simulink model "GolfSwing"  (R2024b)
settings: Solver=VariableStepAuto  StartTime=0.0  StopTime=StopTime  MaxStep=0.001  RelTol=1e-3
PreLoadFcn:
  | cd(matlabdrive);
  | cd '2DModel';
PostLoadFcn:
  | %run SCRIPT_mdlWksGenerate.m;
  | mdlWks=get_param('GolfSwing','ModelWorkspace');
  | mdlWks.DataSource = 'MAT-File';
  | mdlWks.FileName = 'ModelInputs.mat';
  | mdlWks.reload;
model workspace: external: MAT-File ModelInputs.mat (data not in the file)
undefined symbols (not defined in the file or in its folder): GlobalGain, HipConstant, HipDampening, HipTimeGain, KillDampFinalValue, KillDampInitialValue, KillswitchFinalValue, KillswitchInitialValue, KillswitchStepTime, LElbowConstant, LElbowDampening, LElbowTimeGain, LScapConstant, LScapDampening, LScapPositionGain, LScapTimeGain, LShoulderConstant, LShoulderDampening, LShoulderTimeGain, LWristConstant, LWristDampening, LWristTimeGain, RElbowConstant, RElbowDampening, RElbowTimeGain, RScapConstant, RScapDampening, RScapPositionGain, RScapTimeGain, RShoulderConstant, RShoulderDampening, RShoulderTimeGain, RWristConstant, RWristDampening, RWristTimeGain, TorsoConstant, TorsoDampening, TorsoPositionGain, TorsoTimeGain, WristGain, X, Y, Z
libraries: nesl_utility x207, sm_lib x106, matrix_library x11, simulink_extras x2, simulink x1
(part 5 of 6)

== system GolfSwing/Right Upper Arm MOF ==
  RS Global Position : Inport
  RE Global Position : Inport  Port=2
  RSonRArmFGlobalIn : Inport  Port=3
  RSonRArmTGlobalIn : Inport  Port=4
  RForearmonRArmFGlobalIn : Inport  Port=5
  RForearmonRArmTGlobalIn : Inport  Port=6
  R Vector Elbow Force on Right Arm : Sum  Inputs=-+
  R Vector Shoulder Force on Right Arm : Sum  Inputs=-+
  RElbowonRArmMOFGlobal : matrix_library/Cross Product
  RElbowonRArmMOFLocal : Product  Multiplication=Matrix(*)
  RSAngularImpulseonArm : Integrator
  RShoulderonRArmMOFGlobal : matrix_library/Cross Product
  RShoulderonRArmMOFLocal : Product  Multiplication=Matrix(*)
  RUACOM : sm_lib/Body Elements/Inertia Sensor  SensorExtent=BodyGroup  SpanWeldJoints=off  ExcludeGroundedBodies=off  MeasurementFrame=World  SenseMass=off  SenseCenterOfMass=on  SenseInertiaMatrix=off  SenseCenteredInertiaMatrix=off  SensePrincipalInertiaMatrix=off  SenseRotationMatrix=off  GraphicType=None  PrincipalInertiaFrameSize=20  GraphicVisPropType=SimpleVisualProperties  GraphicDiffuseColor=[0.5 0.5 0.5]  GraphicOpacity=1  GraphicSpecularColor=[0.5 0.5 0.5 1.0]  GraphicAmbientColor=[0.15 0.15 0.15 1.0]  GraphicEmissiveColor=[0.0 0.0 0.0 1.0]  GraphicShininess=75
  Right Upper Arm COM : nesl_utility/PS-Simulink Converter  PhysicalDomain=network_engine_domain  SubClassName=ps_output  LeftPortType=input  RightPortType=output  PseudoPeriodic=off  Frequencies=[]  VectorFormat=1-D array  Unit=inherit  AffineConversion=off
  Rotation Transform Right Arm : nesl_utility/PS-Simulink Converter  PhysicalDomain=network_engine_domain  SubClassName=ps_output  LeftPortType=input  RightPortType=output  PseudoPeriodic=off  Frequencies=[]  VectorFormat=1-D array  Unit=inherit  AffineConversion=off
  SumofMomentsRArmLocal : Product  Multiplication=Matrix(*)
  SumofMomentsRSonRArm : Sum
  SumofMomentsRightArmGlobal : Sum  Inputs=++++
  Transform Sensor : sm_lib/Frames and Transforms/Transform Sensor  MeasurementFrame=World  RotationSequence=XYX  SenseAngle=off  SenseAxis=off  SenseQ=off  SenseR=on  SenseRotationSequence=off  SenseOmegaX=off  SenseOmegaY=off  SenseOmegaZ=off  SenseOmega=off  SenseQDot=off  SenseRDot=off  SenseRotationSequenceDot=off  SenseAlphaX=off  SenseAlphaY=off  SenseAlphaZ=off  SenseAlpha=off  SenseQDDot=off  SenseRDDot=off  SenseX=off  SenseY=off  SenseZ=off  SenseXYZ=off  SenseRad=off  SenseAzim=off  SenseDist=off  SenseInc=off  SenseXDot=off  SenseYDot=off  SenseZDot=off  SenseXYZDot=off  SenseRadDot=off  SenseAzimDot=off  SenseDistDot=off  SenseIncDot=off  SenseXDDot=off  SenseYDDot=off  SenseZDDot=off  SenseXYZDDot=off  SenseRadDDot=off  SenseAzimDDot=off  SenseDistDDot=off  SenseIncDDot=off
  World Frame : sm_lib/Frames and Transforms/World Frame
  RightUpper  Arm : PMIOPort  Side=Left
  wires:
  Right Upper Arm COM/1 -> R Vector Elbow Force on Right Arm/1, R Vector Shoulder Force on Right Arm/1  "RUpperArmCOM"
  RS Global Position/1 -> R Vector Shoulder Force on Right Arm/2
  RE Global Position/1 -> R Vector Elbow Force on Right Arm/2
  RSonRArmFGlobalIn/1 -> RShoulderonRArmMOFGlobal/2
  R Vector Elbow Force on Right Arm/1 -> RElbowonRArmMOFGlobal/1
  RForearmonRArmTGlobalIn/1 -> SumofMomentsRightArmGlobal/4
  RForearmonRArmFGlobalIn/1 -> RElbowonRArmMOFGlobal/2
  R Vector Shoulder Force on Right Arm/1 -> RShoulderonRArmMOFGlobal/1
  SumofMomentsRightArmGlobal/1 -> SumofMomentsRArmLocal/2  "SumofMomentsRightArmGlobal"
  RElbowonRArmMOFGlobal/1 -> RElbowonRArmMOFLocal/2, SumofMomentsRightArmGlobal/2  "RElbowonRArmMOFGlobal"
  Rotation Transform Right Arm/1 -> SumofMomentsRArmLocal/1, RElbowonRArmMOFLocal/1, RShoulderonRArmMOFLocal/1
  RShoulderonRArmMOFGlobal/1 -> SumofMomentsRightArmGlobal/1, SumofMomentsRSonRArm/2, RShoulderonRArmMOFLocal/2  "RShoulderonRArmMOFGlobal"
  SumofMomentsRSonRArm/1 -> RSAngularImpulseonArm/1  "SumofMomentsRSonRArm"
  RSonRArmTGlobalIn/1 -> SumofMomentsRSonRArm/1, SumofMomentsRightArmGlobal/3
  connections:
  RUACOM/LConn1 -- Transform Sensor/LConn1 -- RightUpper  Arm/RConn1
  Right Upper Arm COM/LConn1 -- RUACOM/RConn1
  Transform Sensor/RConn1 -- World Frame/RConn1
  Rotation Transform Right Arm/LConn1 -- Transform Sensor/RConn2

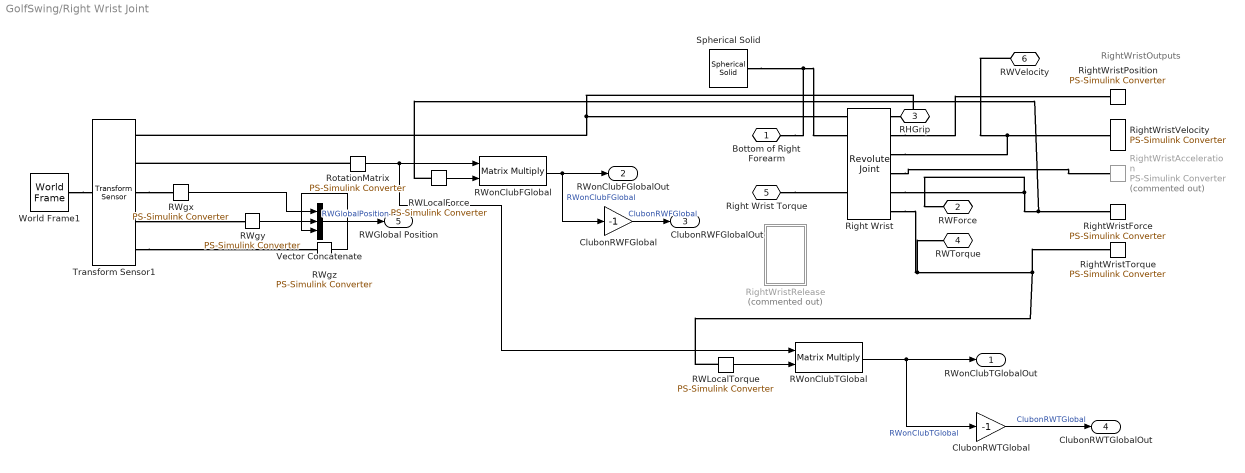
== system GolfSwing/Right Wrist Joint ==
  note: RightWristOutputs
  ClubonRWFGlobal : Gain  Gain=-1
  ClubonRWTGlobal : Gain  Gain=-1
  RWLocalForce : nesl_utility/PS-Simulink Converter  PhysicalDomain=network_engine_domain  SubClassName=ps_output  LeftPortType=input  RightPortType=output  PseudoPeriodic=off  Frequencies=[]  VectorFormat=1-D array  Unit=inherit  AffineConversion=off
  RWLocalTorque : nesl_utility/PS-Simulink Converter  PhysicalDomain=network_engine_domain  SubClassName=ps_output  LeftPortType=input  RightPortType=output  PseudoPeriodic=off  Frequencies=[]  VectorFormat=1-D array  Unit=inherit  AffineConversion=off
  RWgx : nesl_utility/PS-Simulink Converter  PhysicalDomain=network_engine_domain  SubClassName=ps_output  LeftPortType=input  RightPortType=output  PseudoPeriodic=off  Frequencies=[]  VectorFormat=1-D array  Unit=inherit  AffineConversion=off
  RWgy : nesl_utility/PS-Simulink Converter  PhysicalDomain=network_engine_domain  SubClassName=ps_output  LeftPortType=input  RightPortType=output  PseudoPeriodic=off  Frequencies=[]  VectorFormat=1-D array  Unit=inherit  AffineConversion=off
  RWgz : nesl_utility/PS-Simulink Converter  PhysicalDomain=network_engine_domain  SubClassName=ps_output  LeftPortType=input  RightPortType=output  PseudoPeriodic=off  Frequencies=[]  VectorFormat=1-D array  Unit=inherit  AffineConversion=off
  RWonClubFGlobal : Product  Multiplication=Matrix(*)
  RWonClubTGlobal : Product  Multiplication=Matrix(*)
  Right Wrist : sm_lib/Joints/Revolute Joint  JointMode=Normal  CompositeWrenchDir=BaseOnFollower  CompositeWrenchFrame=FollowerFrame  SenseConstraintForce=off  SenseConstraintTorque=off  SenseTotalForce=on  SenseTotalTorque=on  PositionTargetSpecify=off  PositionTargetPriority=Low  PositionTargetValue=70  PositionTargetValueUnits=deg  VelocityTargetSpecify=off  VelocityTargetPriority=Low  VelocityTargetValue=0  VelocityTargetValueUnits=deg/s  EquilibriumPosition=0  EquilibriumPositionUnits=deg  SpringStiffness=0  SpringStiffnessUnits=N*m/deg  DampingCoefficient=0  DampingCoefficientUnits=N*m/(deg/s)  LowerLimitSpecify=off  LowerLimitBound=-90  LowerLimitBoundUnits=deg  LowerLimitStiffness=1e4  LowerLimitStiffnessUnits=N*m/deg  LowerLimitDamping=10  LowerLimitDampingUnits=N*m/(deg/s)  LowerLimitTransitionRegionWidth=0.1  LowerLimitTransitionRegionWidthUnits=deg  UpperLimitSpecify=off  UpperLimitBound=90  UpperLimitBoundUnits=deg  UpperLimitStiffness=1e4  UpperLimitStiffnessUnits=N*m/deg  UpperLimitDamping=10  UpperLimitDampingUnits=N*m/(deg/s)  UpperLimitTransitionRegionWidth=0.1  UpperLimitTransitionRegionWidthUnits=deg  TorqueActuationMode=InputTorque  MotionActuationMode=ComputedMotion  SensePosition=on  SenseVelocity=on  SenseAcceleration=on  SenseTorqueForce=off  SenseLowerLimitTorqueForce=off  SenseUpperLimitTorqueForce=off
      settings: LogSimulationData=on
  RightWristAcceleration : nesl_utility/PS-Simulink Converter  Commented=on  PhysicalDomain=network_engine_domain  SubClassName=ps_output  LeftPortType=input  RightPortType=output  PseudoPeriodic=off  Frequencies=[]  VectorFormat=1-D array  Unit=inherit  AffineConversion=off
  RightWristForce : nesl_utility/PS-Simulink Converter  PhysicalDomain=network_engine_domain  SubClassName=ps_output  LeftPortType=input  RightPortType=output  PseudoPeriodic=off  Frequencies=[]  VectorFormat=1-D array  Unit=inherit  AffineConversion=off
  RightWristPosition : nesl_utility/PS-Simulink Converter  PhysicalDomain=network_engine_domain  SubClassName=ps_output  LeftPortType=input  RightPortType=output  PseudoPeriodic=off  Frequencies=[]  VectorFormat=1-D array  Unit=inherit  AffineConversion=off
  RightWristRelease : Subsystem  Commented=on
  RightWristTorque : nesl_utility/PS-Simulink Converter  PhysicalDomain=network_engine_domain  SubClassName=ps_output  LeftPortType=input  RightPortType=output  PseudoPeriodic=off  Frequencies=[]  VectorFormat=1-D array  Unit=inherit  AffineConversion=off
  RightWristVelocity : nesl_utility/PS-Simulink Converter  PhysicalDomain=network_engine_domain  SubClassName=ps_output  LeftPortType=input  RightPortType=output  PseudoPeriodic=off  Frequencies=[]  VectorFormat=1-D array  Unit=inherit  AffineConversion=off
  RotationMatrix : nesl_utility/PS-Simulink Converter  PhysicalDomain=network_engine_domain  SubClassName=ps_output  LeftPortType=input  RightPortType=output  PseudoPeriodic=off  Frequencies=[]  VectorFormat=1-D array  Unit=inherit  AffineConversion=off
  Spherical Solid : sm_lib/Body Elements/Spherical Solid  SphereRadius=2  SphereRadiusUnits=in  ExportEntireGeometry=off  InertiaType=CalculateFromGeometry  BasedOnType=Density  Density=0  DensityUnits=kg/m^3  Mass=1  MassUnits=kg  CenterOfMass=[0 0 0]  CenterOfMassUnits=m  MomentsOfInertia=[1 1 1]  MomentsOfInertiaUnits=kg*m^2  ProductsOfInertia=[0 0 0]  ProductsOfInertiaUnits=kg*m^2  GraphicType=FromGeometry  MarkerShape=Sphere  MarkerSize=10  GraphicVisPropType=SimpleVisualProperties  GraphicDiffuseColor=[1.0 0.8 0.4]  GraphicOpacity=1  GraphicSpecularColor=[0.5 0.5 0.5 1.0]  GraphicAmbientColor=[0.15 0.15 0.15 1.0]  GraphicEmissiveColor=[0.0 0.0 0.0 1.0]  GraphicShininess=75  DoExposeReferenceFrame=on  SerializedFrames=<Frames/>
  Transform Sensor1 : sm_lib/Frames and Transforms/Transform Sensor  MeasurementFrame=World  RotationSequence=XYX  SenseAngle=off  SenseAxis=off  SenseQ=off  SenseR=on  SenseRotationSequence=off  SenseOmegaX=off  SenseOmegaY=off  SenseOmegaZ=off  SenseOmega=off  SenseQDot=off  SenseRDot=off  SenseRotationSequenceDot=off  SenseAlphaX=off  SenseAlphaY=off  SenseAlphaZ=off  SenseAlpha=off  SenseQDDot=off  SenseRDDot=off  SenseX=on  SenseY=on  SenseZ=on  SenseXYZ=off  SenseRad=off  SenseAzim=off  SenseDist=off  SenseInc=off  SenseXDot=off  SenseYDot=off  SenseZDot=off  SenseXYZDot=off  SenseRadDot=off  SenseAzimDot=off  SenseDistDot=off  SenseIncDot=off  SenseXDDot=off  SenseYDDot=off  SenseZDDot=off  SenseXYZDDot=off  SenseRadDDot=off  SenseAzimDDot=off  SenseDistDDot=off  SenseIncDDot=off
  Vector Concatenate : Concatenate  NumInputs=3
  World Frame1 : sm_lib/Frames and Transforms/World Frame
  Bottom of Right Forearm : PMIOPort  Side=Left
  RWForce : PMIOPort  Port=2  Side=Right
  RHGrip : PMIOPort  Port=3  Side=Right
  RWTorque : PMIOPort  Port=4  Side=Right
  Right Wrist Torque : PMIOPort  Port=5  Side=Right
  RWVelocity : PMIOPort  Port=6  Side=Right
  RWonClubTGlobalOut : Outport
  RWonClubFGlobalOut : Outport  Port=2
  ClubonRWFGlobalOut : Outport  Port=3
  ClubonRWTGlobalOut : Outport  Port=4
  RWGlobal Position : Outport  Port=5
  wires:
  RWLocalForce/1 -> RWonClubFGlobal/2
  RotationMatrix/1 -> RWonClubTGlobal/1, RWonClubFGlobal/1
  RWLocalTorque/1 -> RWonClubTGlobal/2
  ClubonRWFGlobal/1 -> ClubonRWFGlobalOut/1  "ClubonRWFGlobal"
  RWonClubFGlobal/1 -> ClubonRWFGlobal/1, RWonClubFGlobalOut/1  "RWonClubFGlobal"
  RWonClubTGlobal/1 -> ClubonRWTGlobal/1, RWonClubTGlobalOut/1  "RWonClubTGlobal"
  ClubonRWTGlobal/1 -> ClubonRWTGlobalOut/1  "ClubonRWTGlobal"
  RWgx/1 -> Vector Concatenate/1
  RWgz/1 -> Vector Concatenate/3
  Vector Concatenate/1 -> RWGlobal Position/1  "RWGlobalPosition"
  RWgy/1 -> Vector Concatenate/2
  connections:
  Bottom of Right Forearm/RConn1 -- Spherical Solid/RConn1 -- Right Wrist/LConn1
  Right Wrist/RConn1 -- Transform Sensor1/RConn1 -- RHGrip/RConn1
  Right Wrist Torque/RConn1 -- Right Wrist/LConn2
  RotationMatrix/LConn1 -- Transform Sensor1/RConn2
  World Frame1/RConn1 -- Transform Sensor1/LConn1
  Transform Sensor1/RConn4 -- RWgy/LConn1
  Transform Sensor1/RConn5 -- RWgz/LConn1
  Transform Sensor1/RConn3 -- RWgx/LConn1
  Right Wrist/RConn3 -- RightWristVelocity/LConn1 -- RWVelocity/RConn1
  Right Wrist/RConn2 -- RightWristPosition/LConn1
  Right Wrist/RConn5 -- RightWristForce/LConn1 -- RWLocalForce/LConn1 -- RWForce/RConn1
  Right Wrist/RConn6 -- RightWristTorque/LConn1 -- RWLocalTorque/LConn1 -- RWTorque/RConn1
  Right Wrist/RConn4 -- RightWristAcceleration/LConn1

== system GolfSwing/TorsoOutputs ==
  TorsoAcceleration : nesl_utility/PS-Simulink Converter  Commented=on  PhysicalDomain=network_engine_domain  SubClassName=ps_output  LeftPortType=input  RightPortType=output  PseudoPeriodic=off  Frequencies=[]  VectorFormat=1-D array  Unit=inherit  AffineConversion=off
  TorsoForce : nesl_utility/PS-Simulink Converter  PhysicalDomain=network_engine_domain  SubClassName=ps_output  LeftPortType=input  RightPortType=output  PseudoPeriodic=off  Frequencies=[]  VectorFormat=1-D array  Unit=inherit  AffineConversion=off
  TorsoPosition : nesl_utility/PS-Simulink Converter  PhysicalDomain=network_engine_domain  SubClassName=ps_output  LeftPortType=input  RightPortType=output  PseudoPeriodic=off  Frequencies=[]  VectorFormat=1-D array  Unit=inherit  AffineConversion=off
  TorsoTorque : nesl_utility/PS-Simulink Converter  PhysicalDomain=network_engine_domain  SubClassName=ps_output  LeftPortType=input  RightPortType=output  PseudoPeriodic=off  Frequencies=[]  VectorFormat=1-D array  Unit=inherit  AffineConversion=off
  TorsoVelocity : nesl_utility/PS-Simulink Converter  PhysicalDomain=network_engine_domain  SubClassName=ps_output  LeftPortType=input  RightPortType=output  PseudoPeriodic=off  Frequencies=[]  VectorFormat=1-D array  Unit=inherit  AffineConversion=off
  TorsPosition : PMIOPort  Side=Left
  TorsVel : PMIOPort  Port=2  Side=Left
  TorsAccel : PMIOPort  Port=3  Side=Left
  TorsForce : PMIOPort  Port=4  Side=Left
  TorsTorque : PMIOPort  Port=5  Side=Left
  connections:
  TorsForce/RConn1 -- TorsoForce/LConn1
  TorsVel/RConn1 -- TorsoVelocity/LConn1
  TorsTorque/RConn1 -- TorsoTorque/LConn1
  TorsAccel/RConn1 -- TorsoAcceleration/LConn1
  TorsPosition/RConn1 -- TorsoPosition/LConn1

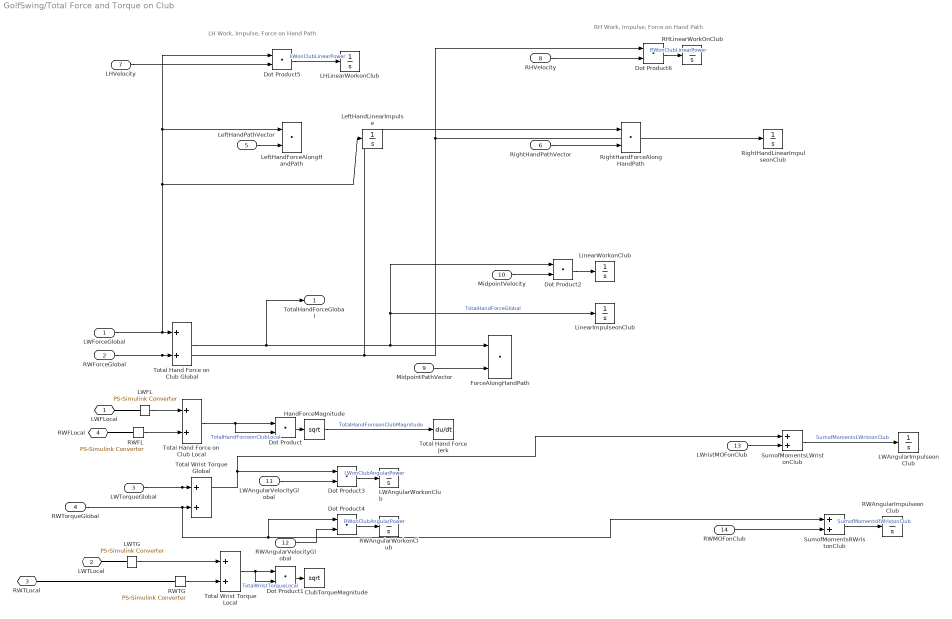
== system GolfSwing/Total Force and Torque on Club ==
  note: RH Work, Impulse, Force on Hand Path
  note: LH Work, Impulse, Force on Hand Path
  LWForceGlobal : Inport
  RWForceGlobal : Inport  Port=2
  LWTorqueGlobal : Inport  Port=3
  RWTorqueGlobal : Inport  Port=4
  LeftHandPathVector : Inport  Port=5
  RightHandPathVector : Inport  Port=6
  LHVelocity : Inport  Port=7
  RHVelocity : Inport  Port=8
  MidpointPathVector : Inport  Port=9
  MidpointVelocity : Inport  Port=10
  LWAngularVelocityGlobal : Inport  Port=11
  RWAngularVelocityGlobal : Inport  Port=12
  LWristMOFonClub : Inport  Port=13
  RWMOFonClub : Inport  Port=14
  ClubTorqueMagnitude : Sqrt
  Dot Product{,1..6} (7 alike) : DotProduct  OutDataTypeStr=Inherit: Inherit via internal rule
  ForceAlongHandPath : DotProduct  OutDataTypeStr=Inherit: Inherit via internal rule
  HandForceMagnitude : Sqrt
  LHLinearWorkonClub : Integrator
  LWAngularImpulseonClub : Integrator
  LWAngularWorkonClub : Integrator
  LWFL : nesl_utility/PS-Simulink Converter  PhysicalDomain=network_engine_domain  SubClassName=ps_output  LeftPortType=input  RightPortType=output  PseudoPeriodic=off  Frequencies=[]  VectorFormat=1-D array  Unit=inherit  AffineConversion=off
  LWTG : nesl_utility/PS-Simulink Converter  PhysicalDomain=network_engine_domain  SubClassName=ps_output  LeftPortType=input  RightPortType=output  PseudoPeriodic=off  Frequencies=[]  VectorFormat=1-D array  Unit=inherit  AffineConversion=off
  LeftHandForceAlongHandPath : DotProduct  OutDataTypeStr=Inherit: Inherit via internal rule
  LeftHandLinearImpulse : Integrator
  LinearImpulseonClub : Integrator
  LinearWorkonClub : Integrator
  RHLinearWorkOnClub : Integrator
  RWAngularImpulseonClub : Integrator
  RWAngularWorkonClub : Integrator
  RWFL : nesl_utility/PS-Simulink Converter  PhysicalDomain=network_engine_domain  SubClassName=ps_output  LeftPortType=input  RightPortType=output  PseudoPeriodic=off  Frequencies=[]  VectorFormat=1-D array  Unit=inherit  AffineConversion=off
  RWTG : nesl_utility/PS-Simulink Converter  PhysicalDomain=network_engine_domain  SubClassName=ps_output  LeftPortType=input  RightPortType=output  PseudoPeriodic=off  Frequencies=[]  VectorFormat=1-D array  Unit=inherit  AffineConversion=off
  RightHandForceAlongHandPath : DotProduct  OutDataTypeStr=Inherit: Inherit via internal rule
  RightHandLinearImpulseonClub : Integrator
  SumofMomentsLWristonClub : Sum
  SumofMomentsRWristonClub : Sum
  Total Hand Force Jerk : Derivative
  Total Hand Force on Club Global : Sum
  Total Hand Force on Club Local : Sum
  Total Wrist Torque Global : Sum
  Total Wrist Torque Local : Sum
  LWFLocal : PMIOPort  Side=Left
  LWTLocal : PMIOPort  Port=2  Side=Left
  RWTLocal : PMIOPort  Port=3  Side=Left
  RWFLocal : PMIOPort  Port=4  Side=Left
  TotalHandForceGlobal : Outport
  wires:
  RWFL/1 -> Total Hand Force on Club Local/2
  Total Wrist Torque Local/1 -> Dot Product1/1, Dot Product1/2  "TotalWristTorqueLocal"
  LWFL/1 -> Total Hand Force on Club Local/1
  Dot Product/1 -> HandForceMagnitude/1
  Dot Product1/1 -> ClubTorqueMagnitude/1
  Total Hand Force on Club Local/1 -> Dot Product/2, Dot Product/1  "TotalHandForceonClubLocal"
  Total Hand Force on Club Global/1 -> Dot Product2/1, LinearImpulseonClub/1, ForceAlongHandPath/1, TotalHandForceGlobal/1  "TotalHandForceGlobal"
  LWTG/1 -> Total Wrist Torque Local/1
  RWTG/1 -> Total Wrist Torque Local/2
  LWTorqueGlobal/1 -> Dot Product3/1, SumofMomentsLWristonClub/1, Total Wrist Torque Global/1
  MidpointPathVector/1 -> ForceAlongHandPath/2
  Dot Product2/1 -> LinearWorkonClub/1
  MidpointVelocity/1 -> Dot Product2/2
  Dot Product3/1 -> LWAngularWorkonClub/1  "LWonClubAngularPower"
  LWAngularVelocityGlobal/1 -> Dot Product3/2
  Dot Product4/1 -> RWAngularWorkonClub/1  "RWonClubAngularPower"
  RWAngularVelocityGlobal/1 -> Dot Product4/2
  RWTorqueGlobal/1 -> Dot Product4/1, SumofMomentsRWristonClub/1, Total Wrist Torque Global/2
  SumofMomentsLWristonClub/1 -> LWAngularImpulseonClub/1  "SumofMomentsLWristonClub"
  SumofMomentsRWristonClub/1 -> RWAngularImpulseonClub/1  "SumofMomentsRWristonClub"
  LWristMOFonClub/1 -> SumofMomentsLWristonClub/2
  RWMOFonClub/1 -> SumofMomentsRWristonClub/2
  LHVelocity/1 -> Dot Product5/2
  LWForceGlobal/1 -> Dot Product5/1, LeftHandForceAlongHandPath/1, LeftHandLinearImpulse/1, Total Hand Force on Club Global/1
  Dot Product5/1 -> LHLinearWorkonClub/1  "LWonClubLinearPower"
  LeftHandPathVector/1 -> LeftHandForceAlongHandPath/2
  RHVelocity/1 -> Dot Product6/2
  RWForceGlobal/1 -> RightHandLinearImpulseonClub/1, Dot Product6/1, RightHandForceAlongHandPath/1, Total Hand Force on Club Global/2
  Dot Product6/1 -> RHLinearWorkOnClub/1  "RWonClubLinearPower"
  RightHandPathVector/1 -> RightHandForceAlongHandPath/2
  HandForceMagnitude/1 -> Total Hand Force Jerk/1  "TotalHandForceonClubMagnitude"
  connections:
  LWFLocal/RConn1 -- LWFL/LConn1
  RWFLocal/RConn1 -- RWFL/LConn1
  LWTG/LConn1 -- LWTLocal/RConn1
  RWTLocal/RConn1 -- RWTG/LConn1

== system GolfSwing/Club/ButtGlobal ==
  Buttx : nesl_utility/PS-Simulink Converter  PhysicalDomain=network_engine_domain  SubClassName=ps_output  LeftPortType=input  RightPortType=output  PseudoPeriodic=off  Frequencies=[]  VectorFormat=1-D array  Unit=inherit  AffineConversion=off
  Butty : nesl_utility/PS-Simulink Converter  PhysicalDomain=network_engine_domain  SubClassName=ps_output  LeftPortType=input  RightPortType=output  PseudoPeriodic=off  Frequencies=[]  VectorFormat=1-D array  Unit=inherit  AffineConversion=off
  Buttz : nesl_utility/PS-Simulink Converter  PhysicalDomain=network_engine_domain  SubClassName=ps_output  LeftPortType=input  RightPortType=output  PseudoPeriodic=off  Frequencies=[]  VectorFormat=1-D array  Unit=inherit  AffineConversion=off
  Transform Sensor : sm_lib/Frames and Transforms/Transform Sensor  MeasurementFrame=World  RotationSequence=XYX  SenseAngle=off  SenseAxis=off  SenseQ=off  SenseR=off  SenseRotationSequence=off  SenseOmegaX=off  SenseOmegaY=off  SenseOmegaZ=off  SenseOmega=off  SenseQDot=off  SenseRDot=off  SenseRotationSequenceDot=off  SenseAlphaX=off  SenseAlphaY=off  SenseAlphaZ=off  SenseAlpha=off  SenseQDDot=off  SenseRDDot=off  SenseX=on  SenseY=on  SenseZ=on  SenseXYZ=off  SenseRad=off  SenseAzim=off  SenseDist=off  SenseInc=off  SenseXDot=off  SenseYDot=off  SenseZDot=off  SenseXYZDot=off  SenseRadDot=off  SenseAzimDot=off  SenseDistDot=off  SenseIncDot=off  SenseXDDot=off  SenseYDDot=off  SenseZDDot=off  SenseXYZDDot=off  SenseRadDDot=off  SenseAzimDDot=off  SenseDistDDot=off  SenseIncDDot=off
  Conn1 : PMIOPort  Side=Right
  Conn2 : PMIOPort  Port=2  Side=Left
  connections:
  Buttx/LConn1 -- Transform Sensor/RConn2
  Buttz/LConn1 -- Transform Sensor/RConn4
  Butty/LConn1 -- Transform Sensor/RConn3
  Transform Sensor/LConn1 -- Conn2/RConn1
  Transform Sensor/RConn1 -- Conn1/RConn1

== system GolfSwing/Club/CHGlobal ==
  AoA Calculation : Subsystem
  CHS (m/s) : Subsystem
  CHSmph : Gain  Gain=2.23694
  CHvx : nesl_utility/PS-Simulink Converter  PhysicalDomain=network_engine_domain  SubClassName=ps_output  LeftPortType=input  RightPortType=output  PseudoPeriodic=off  Frequencies=[]  VectorFormat=1-D array  Unit=inherit  AffineConversion=off
  CHvy : nesl_utility/PS-Simulink Converter  PhysicalDomain=network_engine_domain  SubClassName=ps_output  LeftPortType=input  RightPortType=output  PseudoPeriodic=off  Frequencies=[]  VectorFormat=1-D array  Unit=inherit  AffineConversion=off
  CHvz : nesl_utility/PS-Simulink Converter  PhysicalDomain=network_engine_domain  SubClassName=ps_output  LeftPortType=input  RightPortType=output  PseudoPeriodic=off  Frequencies=[]  VectorFormat=1-D array  Unit=inherit  AffineConversion=off
  CHx : nesl_utility/PS-Simulink Converter  PhysicalDomain=network_engine_domain  SubClassName=ps_output  LeftPortType=input  RightPortType=output  PseudoPeriodic=off  Frequencies=[]  VectorFormat=1-D array  Unit=inherit  AffineConversion=off
  CHy : nesl_utility/PS-Simulink Converter  PhysicalDomain=network_engine_domain  SubClassName=ps_output  LeftPortType=input  RightPortType=output  PseudoPeriodic=off  Frequencies=[]  VectorFormat=1-D array  Unit=inherit  AffineConversion=off
  CHz : nesl_utility/PS-Simulink Converter  PhysicalDomain=network_engine_domain  SubClassName=ps_output  LeftPortType=input  RightPortType=output  PseudoPeriodic=off  Frequencies=[]  VectorFormat=1-D array  Unit=inherit  AffineConversion=off
  ClubheadPathUnitVector : Mux  Inputs=3
  Constant : Constant  Value=0
  Filtering Block : Subsystem  Commented=on
  MinMax Running Resettable : simulink/Math Operations/MinMax Running Resettable  Function=max  vinit=0.0
  Path Calculation : Subsystem
  Transform Sensor : sm_lib/Frames and Transforms/Transform Sensor  MeasurementFrame=World  RotationSequence=XYX  SenseAngle=off  SenseAxis=off  SenseQ=off  SenseR=off  SenseRotationSequence=off  SenseOmegaX=off  SenseOmegaY=off  SenseOmegaZ=off  SenseOmega=off  SenseQDot=off  SenseRDot=off  SenseRotationSequenceDot=off  SenseAlphaX=off  SenseAlphaY=off  SenseAlphaZ=off  SenseAlpha=off  SenseQDDot=off  SenseRDDot=off  SenseX=on  SenseY=on  SenseZ=on  SenseXYZ=off  SenseRad=off  SenseAzim=off  SenseDist=off  SenseInc=off  SenseXDot=on  SenseYDot=on  SenseZDot=on  SenseXYZDot=off  SenseRadDot=off  SenseAzimDot=off  SenseDistDot=off  SenseIncDot=off  SenseXDDot=off  SenseYDDot=off  SenseZDDot=off  SenseXYZDDot=off  SenseRadDDot=off  SenseAzimDDot=off  SenseDistDDot=off  SenseIncDDot=off
  UnitVectorX : Product  Inputs=*/
  UnitVectorY : Product  Inputs=*/
  UnitVectorZ : Product  Inputs=*/
  Clubhead : PMIOPort  Side=Right
  Global : PMIOPort  Port=2  Side=Left
  ClubPathUV : Outport
  CHSMPS : Outport  Port=2
  wires:
  CHvy/1 -> Path Calculation/1(Vy), AoA Calculation/2(Vy), UnitVectorY/1, CHS (m/s)/2(In2)  "CHvy"
  CHvx/1 -> AoA Calculation/1(Vx), Path Calculation/2(Vx), UnitVectorX/1, CHS (m/s)/1(In1)  "CHvx"
  CHvz/1 -> CHS (m/s)/3(In3), AoA Calculation/3(Vz), UnitVectorZ/1  "CHvz"
  UnitVectorZ/1 -> ClubheadPathUnitVector/3
  UnitVectorY/1 -> ClubheadPathUnitVector/2
  CHS (m/s)/1(ClubPathUV1) -> CHSMPS/1, CHSmph/1, UnitVectorZ/2, UnitVectorY/2, UnitVectorX/2  "CHSmpersec"
  UnitVectorX/1 -> ClubheadPathUnitVector/1
  ClubheadPathUnitVector/1 -> ClubPathUV/1  "ClubPathUV"
  CHSmph/1 -> MinMax Running Resettable/1, Filtering Block/1(CHS (mph))  "CHS (mph)"
  Constant/1 -> MinMax Running Resettable/2
  connections:
  CHx/LConn1 -- Transform Sensor/RConn2
  CHz/LConn1 -- Transform Sensor/RConn4
  CHvz/LConn1 -- Transform Sensor/RConn7
  CHy/LConn1 -- Transform Sensor/RConn3
  Transform Sensor/RConn5 -- CHvx/LConn1
  CHvy/LConn1 -- Transform Sensor/RConn6
  Transform Sensor/LConn1 -- Global/RConn1
  Transform Sensor/RConn1 -- Clubhead/RConn1

== system GolfSwing/Club/Clubhead Air Resistance Calculator ==
  CHSmps : Inport
  ClubPathUV : Inport  Port=2
  Add : Sum  Inputs=+++
  Air Resistance : sm_lib/Forces and Torques/External Force and Torque  EnableForceX=off  EnableForceY=off  EnableForceZ=off  EnableForce=on  ForceResolutionFrame=World  EnableTorqueX=off  EnableTorqueY=off  EnableTorqueZ=off  EnableTorque=off  TorqueResolutionFrame=AttachedFrame
  Demux : Demux  Outputs=3
  Drag Function : MATLAB Function  TreatAsAtomicUnit=on
  Math Function : Math  Operator=square
  Math Function1 : Math  Operator=square
  Math Function2 : Math  Operator=square
  Matrix Multiply : Product
  Simulink-PS Converter : nesl_utility/Simulink-PS Converter  PhysicalDomain=network_engine_domain  SubClassName=ps_input  LeftPortType=input  RightPortType=output  PseudoPeriodic=off  Frequencies=[]  NoiseDistribution=none  NoiseParameters=[]  Unit=1  AffineConversion=off  FilteringAndDerivatives=provide  SimscapeFilterOrder=1  InputFilterTimeConstant=0.001  UdotUserProvided=0
  Sqrt : Sqrt
  FDrag : PMIOPort  Side=Right
  wires:
  ClubPathUV/1 -> Matrix Multiply/2
  Matrix Multiply/1 -> Demux/1, Simulink-PS Converter/1  "FDrag"
  CHSmps/1 -> Drag Function/1(u)
  Drag Function/1(FDrag) -> Matrix Multiply/1
  Add/1 -> Sqrt/1
  Math Function2/1 -> Add/3
  Math Function/1 -> Add/1
  Math Function1/1 -> Add/2
  Demux/2 -> Math Function1/1
  Demux/1 -> Math Function/1
  Demux/3 -> Math Function2/1
  connections:
  Air Resistance/RConn1 -- FDrag/RConn1
  Simulink-PS Converter/RConn1 -- Air Resistance/LConn1

== system GolfSwing/Club/Flexible Beam Model ==
  Flexible Cylindrical Beam : sm_lib/Body Elements/Flexible Bodies/Beams/Flexible Cylindrical Beam  SectionType=Hollow  Radius=0.010  RadiusUnits=m  Thickness=0.0015  ThicknessUnits=m  Length=ShaftLength  LengthUnits=m  StiffnessAndInertiaType=CalculateFromGeometry  Density=500  DensityUnits=kg/m^3  ModuliType=YoungsPoissons  YoungsModulus=ShaftStiffness  YoungsModulusUnits=GPa  PoissonsRatio=0.33  ShearModulus=26  ShearModulusUnits=GPa  GeometricCentroid=[0 0]  GeometricCentroidUnits=m  BendingCentroid=[0 0]  BendingCentroidUnits=m  ShearCenter=[0 0]  ShearCenterUnits=m  AxialRigidity=1  AxialRigidityUnits=Pa*m^2  FlexuralRigidity=[1 1]  FlexuralRigidityUnits=Pa*m^4  CrossFlexuralRigidity=0  CrossFlexuralRigidityUnits=Pa*m^4  TorsionalRigidity=1  TorsionalRigidityUnits=Pa*m^4  CenterOfMass=[0 0]  CenterOfMassUnits=m  MassPerUnitLength=1  MassPerUnitLengthUnits=kg/m  MassMomentOfInertiaDensity=[1 1]  MassMomentOfInertiaDensityUnits=kg*m  MassProductOfInertiaDensity=0  MassProductOfInertiaDensityUnits=kg*m  DampingType=Proportional  ProportionalDampingAlpha=0  ProportionalDampingAlphaUnits=1/s  ProportionalDampingBeta=ShaftDampening  ProportionalDampingBetaUnits=s  UniformModalDampingRatio=0.01  NumElements=1  ReductionType=None  NumRetainedModes=1  GraphicType=FromGeometry  GraphicVisPropType=SimpleVisualProperties  GraphicDiffuseColor=[0.5 0.5 0.5]  GraphicOpacity=1.0  GraphicSpecularColor=[0.5 0.5 0.5 1.0]  GraphicAmbientColor=[0.15 0.15 0.15 1.0]  GraphicEmissiveColor=[0.0 0.0 0.0 1.0]  GraphicShininess=75  DoExposeZminFrame=on  DoExposeZmaxFrame=on  SerializedFrames=<Frames/>
  Rigid Transform : sm_lib/Frames and Transforms/Rigid Transform  RotationMethod=RotationSequence  FollAlignAxisA=+X  BaseAlignAxisA=+Y  FollAlignAxisB=+Y  BaseAlignAxisB=+Z  RotationStandardAxis=+Z  RotationAngle=0.0  RotationAngleUnits=deg  RotationArbitraryAxis=[0 0 1]  RotationSequenceAxes=FollowerAxes  RotationSequence=XYX  RotationSequenceAngles=[0 90 0]  RotationSequenceAnglesUnits=deg  RotationMatrix=[1 0 0; 0 1 0; 0 0 1]  Quaternion=[1 0 0 0]  TranslationMethod=None  TranslationCartesianOffset=[0 0 0]  TranslationCartesianOffsetUnits=m  TranslationStandardAxis=+Z  TranslationStandardOffset=0  TranslationStandardOffsetUnits=m  TranslationROffset=0  TranslationROffsetUnits=m  TranslationThetaOffset=0  TranslationThetaOffsetUnits=deg  TranslationZOffset=0  TranslationZOffsetUnits=m
  RH Grip : PMIOPort  Side=Left
  Clubhead : PMIOPort  Port=2  Side=Right
  connections:
  Rigid Transform/RConn1 -- Flexible Cylindrical Beam/LConn1
  RH Grip/RConn1 -- Rigid Transform/LConn1
  Flexible Cylindrical Beam/RConn1 -- Clubhead/RConn1

== system GolfSwing/Club/Impact Model ==
  CHSmps : Inport
  ClubPathUV : Inport  Port=2
  Add1 : Sum
  Golf Ball Reaction Force : MATLAB Function  TreatAsAtomicUnit=on
  Golf Ball Rxn Force : sm_lib/Forces and Torques/External Force and Torque  EnableForceX=off  EnableForceY=off  EnableForceZ=off  EnableForce=on  ForceResolutionFrame=World  EnableTorqueX=off  EnableTorqueY=off  EnableTorqueZ=off  EnableTorque=off  TorqueResolutionFrame=AttachedFrame
  Matrix Multiply : Product
  Matrix Multiply1 : Product
  Simulink-PS Converter : nesl_utility/Simulink-PS Converter  PhysicalDomain=network_engine_domain  SubClassName=ps_input  LeftPortType=input  RightPortType=output  PseudoPeriodic=off  Frequencies=[]  NoiseDistribution=none  NoiseParameters=[]  Unit=1  AffineConversion=off  FilteringAndDerivatives=provide  SimscapeFilterOrder=1  InputFilterTimeConstant=0.001  UdotUserProvided=0
  Step : Step  Time=0.24  SampleTime=0
  Step1 : Step  Time=0.2405  After=-1  SampleTime=0
  FBRxn : PMIOPort  Side=Right
  wires:
  ClubPathUV/1 -> Matrix Multiply/2
  Matrix Multiply/1 -> Simulink-PS Converter/1  "FImpact"
  CHSmps/1 -> Golf Ball Reaction Force/1(u)
  Step1/1 -> Add1/2
  Step/1 -> Add1/1
  Add1/1 -> Matrix Multiply1/1
  Golf Ball Reaction Force/1(FImpact) -> Matrix Multiply1/2
  Matrix Multiply1/1 -> Matrix Multiply/1  "FImpactMag"
  connections:
  Golf Ball Rxn Force/RConn1 -- FBRxn/RConn1
  Simulink-PS Converter/RConn1 -- Golf Ball Rxn Force/LConn1

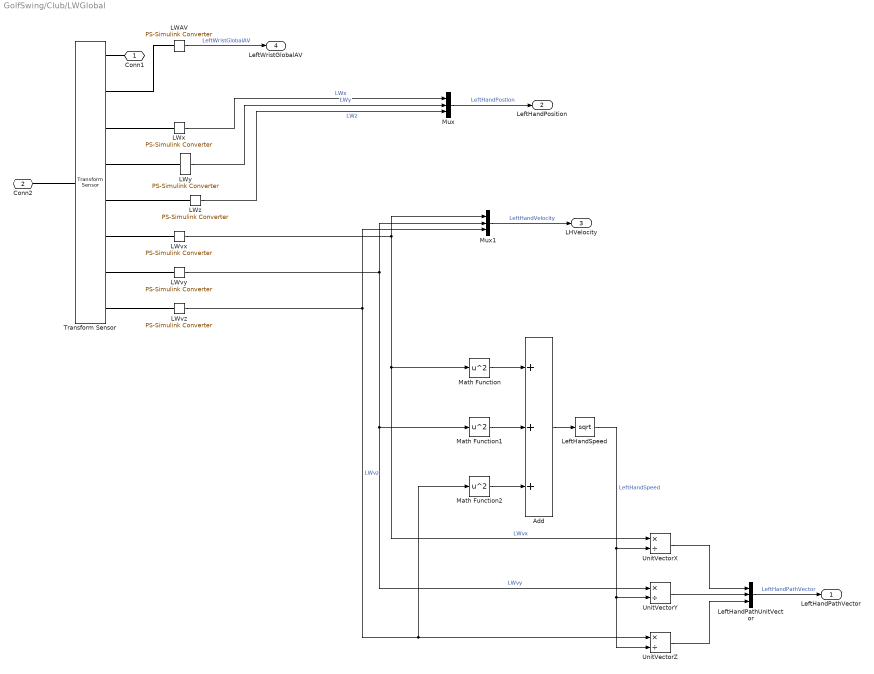
== system GolfSwing/Club/LWGlobal ==
  Add : Sum  Inputs=+++
  LWAV : nesl_utility/PS-Simulink Converter  PhysicalDomain=network_engine_domain  SubClassName=ps_output  LeftPortType=input  RightPortType=output  PseudoPeriodic=off  Frequencies=[]  VectorFormat=1-D array  Unit=inherit  AffineConversion=off
  LWvx : nesl_utility/PS-Simulink Converter  PhysicalDomain=network_engine_domain  SubClassName=ps_output  LeftPortType=input  RightPortType=output  PseudoPeriodic=off  Frequencies=[]  VectorFormat=1-D array  Unit=inherit  AffineConversion=off
  LWvy : nesl_utility/PS-Simulink Converter  PhysicalDomain=network_engine_domain  SubClassName=ps_output  LeftPortType=input  RightPortType=output  PseudoPeriodic=off  Frequencies=[]  VectorFormat=1-D array  Unit=inherit  AffineConversion=off
  LWvz : nesl_utility/PS-Simulink Converter  PhysicalDomain=network_engine_domain  SubClassName=ps_output  LeftPortType=input  RightPortType=output  PseudoPeriodic=off  Frequencies=[]  VectorFormat=1-D array  Unit=inherit  AffineConversion=off
  LWx : nesl_utility/PS-Simulink Converter  PhysicalDomain=network_engine_domain  SubClassName=ps_output  LeftPortType=input  RightPortType=output  PseudoPeriodic=off  Frequencies=[]  VectorFormat=1-D array  Unit=inherit  AffineConversion=off
  LWy : nesl_utility/PS-Simulink Converter  PhysicalDomain=network_engine_domain  SubClassName=ps_output  LeftPortType=input  RightPortType=output  PseudoPeriodic=off  Frequencies=[]  VectorFormat=1-D array  Unit=inherit  AffineConversion=off
  LWz : nesl_utility/PS-Simulink Converter  PhysicalDomain=network_engine_domain  SubClassName=ps_output  LeftPortType=input  RightPortType=output  PseudoPeriodic=off  Frequencies=[]  VectorFormat=1-D array  Unit=inherit  AffineConversion=off
  LeftHandPathUnitVector : Mux  Inputs=3
  LeftHandSpeed : Sqrt
  Math Function : Math  Operator=square
  Math Function1 : Math  Operator=square
  Math Function2 : Math  Operator=square
  Mux : Mux  Inputs=3
  Mux1 : Mux  Inputs=3
  Transform Sensor : sm_lib/Frames and Transforms/Transform Sensor  MeasurementFrame=World  RotationSequence=XYX  SenseAngle=off  SenseAxis=off  SenseQ=off  SenseR=off  SenseRotationSequence=off  SenseOmegaX=off  SenseOmegaY=off  SenseOmegaZ=off  SenseOmega=on  SenseQDot=off  SenseRDot=off  SenseRotationSequenceDot=off  SenseAlphaX=off  SenseAlphaY=off  SenseAlphaZ=off  SenseAlpha=off  SenseQDDot=off  SenseRDDot=off  SenseX=on  SenseY=on  SenseZ=on  SenseXYZ=off  SenseRad=off  SenseAzim=off  SenseDist=off  SenseInc=off  SenseXDot=on  SenseYDot=on  SenseZDot=on  SenseXYZDot=off  SenseRadDot=off  SenseAzimDot=off  SenseDistDot=off  SenseIncDot=off  SenseXDDot=off  SenseYDDot=off  SenseZDDot=off  SenseXYZDDot=off  SenseRadDDot=off  SenseAzimDDot=off  SenseDistDDot=off  SenseIncDDot=off
  UnitVectorX : Product  Inputs=*/
  UnitVectorY : Product  Inputs=*/
  UnitVectorZ : Product  Inputs=*/
  Conn1 : PMIOPort  Side=Right
  Conn2 : PMIOPort  Port=2  Side=Left
  LeftHandPathVector : Outport
  LeftHandPosition : Outport  Port=2
  LHVelocity : Outport  Port=3
  LeftWristGlobalAV : Outport  Port=4
  wires:
  LWx/1 -> Mux/1  "LWx"
  LWy/1 -> Mux/2  "LWy"
  LWz/1 -> Mux/3  "LWz"
  UnitVectorZ/1 -> LeftHandPathUnitVector/3
  UnitVectorY/1 -> LeftHandPathUnitVector/2
  LeftHandPathUnitVector/1 -> LeftHandPathVector/1  "LeftHandPathVector"
  UnitVectorX/1 -> LeftHandPathUnitVector/1
  Add/1 -> LeftHandSpeed/1
  Math Function/1 -> Add/1
  Math Function1/1 -> Add/2
  Math Function2/1 -> Add/3
  LWvy/1 -> UnitVectorY/1, Math Function1/1, Mux1/2  "LWvy"
  LeftHandSpeed/1 -> UnitVectorX/2, UnitVectorY/2, UnitVectorZ/2  "LeftHandSpeed"
  LWvz/1 -> Mux1/3, Math Function2/1, UnitVectorZ/1  "LWvz"
  LWvx/1 -> Mux1/1, UnitVectorX/1, Math Function/1  "LWvx"
  Mux/1 -> LeftHandPosition/1  "LeftHandPostion"
  Mux1/1 -> LHVelocity/1  "LeftHandVelocity"
  LWAV/1 -> LeftWristGlobalAV/1  "LeftWristGlobalAV"
  connections:
  LWx/LConn1 -- Transform Sensor/RConn3
  LWz/LConn1 -- Transform Sensor/RConn5
  LWvz/LConn1 -- Transform Sensor/RConn8
  LWy/LConn1 -- Transform Sensor/RConn4
  LWvx/LConn1 -- Transform Sensor/RConn6
  LWvy/LConn1 -- Transform Sensor/RConn7
  Transform Sensor/LConn1 -- Conn2/RConn1
  Transform Sensor/RConn1 -- Conn1/RConn1
  LWAV/LConn1 -- Transform Sensor/RConn2

== system GolfSwing/Club/MidpointGlobal ==
  Add : Sum  Inputs=+++
  Hand Speed (mph) : Gain  Gain=2.23694
  MPvx : nesl_utility/PS-Simulink Converter  PhysicalDomain=network_engine_domain  SubClassName=ps_output  LeftPortType=input  RightPortType=output  PseudoPeriodic=off  Frequencies=[]  VectorFormat=1-D array  Unit=inherit  AffineConversion=off
  MPvy : nesl_utility/PS-Simulink Converter  PhysicalDomain=network_engine_domain  SubClassName=ps_output  LeftPortType=input  RightPortType=output  PseudoPeriodic=off  Frequencies=[]  VectorFormat=1-D array  Unit=inherit  AffineConversion=off
  MPvz : nesl_utility/PS-Simulink Converter  PhysicalDomain=network_engine_domain  SubClassName=ps_output  LeftPortType=input  RightPortType=output  PseudoPeriodic=off  Frequencies=[]  VectorFormat=1-D array  Unit=inherit  AffineConversion=off
  MPx : nesl_utility/PS-Simulink Converter  PhysicalDomain=network_engine_domain  SubClassName=ps_output  LeftPortType=input  RightPortType=output  PseudoPeriodic=off  Frequencies=[]  VectorFormat=1-D array  Unit=inherit  AffineConversion=off
  MPy : nesl_utility/PS-Simulink Converter  PhysicalDomain=network_engine_domain  SubClassName=ps_output  LeftPortType=input  RightPortType=output  PseudoPeriodic=off  Frequencies=[]  VectorFormat=1-D array  Unit=inherit  AffineConversion=off
  MPz : nesl_utility/PS-Simulink Converter  PhysicalDomain=network_engine_domain  SubClassName=ps_output  LeftPortType=input  RightPortType=output  PseudoPeriodic=off  Frequencies=[]  VectorFormat=1-D array  Unit=inherit  AffineConversion=off
  Math Function : Math  Operator=square
  Math Function1 : Math  Operator=square
  Math Function2 : Math  Operator=square
  MidHandPathUnitVector : Mux  Inputs=3
  MidHandSpeed : Sqrt
  MidpointAV : nesl_utility/PS-Simulink Converter  PhysicalDomain=network_engine_domain  SubClassName=ps_output  LeftPortType=input  RightPortType=output  PseudoPeriodic=off  Frequencies=[]  VectorFormat=1-D array  Unit=inherit  AffineConversion=off
  Mux : Mux  Inputs=3
  Mux1 : Mux  Inputs=3
  Transform Sensor : sm_lib/Frames and Transforms/Transform Sensor  MeasurementFrame=World  RotationSequence=XYX  SenseAngle=off  SenseAxis=off  SenseQ=off  SenseR=off  SenseRotationSequence=off  SenseOmegaX=off  SenseOmegaY=off  SenseOmegaZ=off  SenseOmega=on  SenseQDot=off  SenseRDot=off  SenseRotationSequenceDot=off  SenseAlphaX=off  SenseAlphaY=off  SenseAlphaZ=off  SenseAlpha=off  SenseQDDot=off  SenseRDDot=off  SenseX=on  SenseY=on  SenseZ=on  SenseXYZ=off  SenseRad=off  SenseAzim=off  SenseDist=off  SenseInc=off  SenseXDot=on  SenseYDot=on  SenseZDot=on  SenseXYZDot=off  SenseRadDot=off  SenseAzimDot=off  SenseDistDot=off  SenseIncDot=off  SenseXDDot=off  SenseYDDot=off  SenseZDDot=off  SenseXYZDDot=off  SenseRadDDot=off  SenseAzimDDot=off  SenseDistDDot=off  SenseIncDDot=off
  UnitVectorX : Product  Inputs=*/
  UnitVectorY : Product  Inputs=*/
  UnitVectorZ : Product  Inputs=*/
  Conn1 : PMIOPort  Side=Right
  Conn2 : PMIOPort  Port=2  Side=Left
  HandPathVector : Outport
  MidHandPosition : Outport  Port=2
  MidHandVelocity : Outport  Port=3
  wires:
  Math Function1/1 -> Add/2
  MidHandSpeed/1 -> UnitVectorZ/2, UnitVectorY/2, UnitVectorX/2, Hand Speed (mph)/1  "MidHandSpeed"
  Math Function/1 -> Add/1
  Math Function2/1 -> Add/3
  Add/1 -> MidHandSpeed/1
  UnitVectorX/1 -> MidHandPathUnitVector/1
  UnitVectorY/1 -> MidHandPathUnitVector/2
  UnitVectorZ/1 -> MidHandPathUnitVector/3
  MidHandPathUnitVector/1 -> HandPathVector/1  "MPPathVector"
  MPy/1 -> Mux/2  "MPy"
  MPz/1 -> Mux/3  "MPz"
  Mux/1 -> MidHandPosition/1  "MidHandPosition"
  MPx/1 -> Mux/1  "MPx"
  MPvy/1 -> Math Function1/1, UnitVectorY/1, Mux1/2  "MPvy"
  MPvz/1 -> Mux1/3, UnitVectorZ/1, Math Function2/1  "MPvz"
  Mux1/1 -> MidHandVelocity/1  "MidHandVelocity"
  MPvx/1 -> Mux1/1, UnitVectorX/1, Math Function/1  "MPvx"
  connections:
  MPx/LConn1 -- Transform Sensor/RConn3
  MPz/LConn1 -- Transform Sensor/RConn5
  MPvz/LConn1 -- Transform Sensor/RConn8
  MPy/LConn1 -- Transform Sensor/RConn4
  MPvx/LConn1 -- Transform Sensor/RConn6
  MPvy/LConn1 -- Transform Sensor/RConn7
  Transform Sensor/LConn1 -- Conn2/RConn1
  Transform Sensor/RConn1 -- Conn1/RConn1
  MidpointAV/LConn1 -- Transform Sensor/RConn2

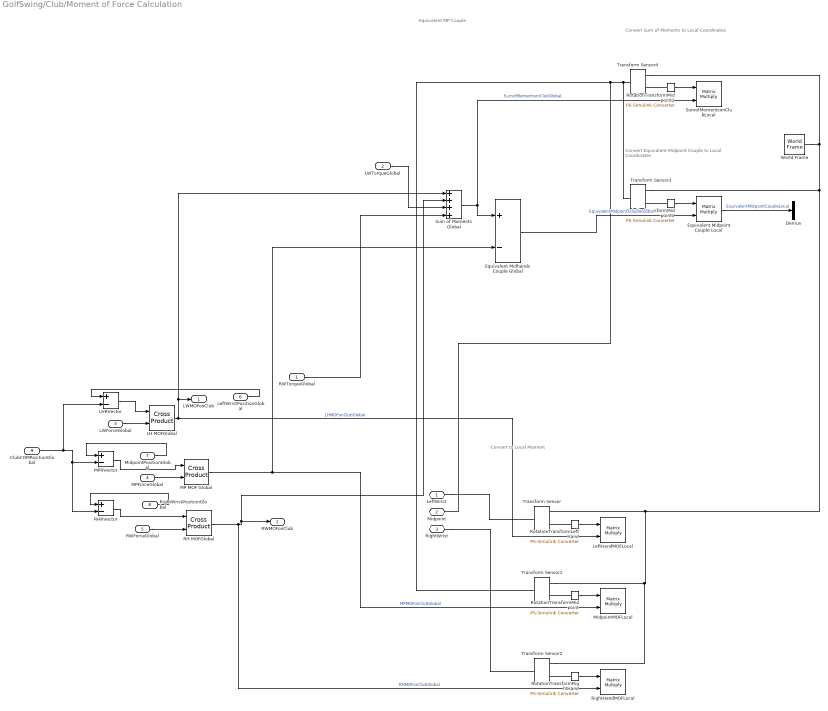
== system GolfSwing/Club/Moment of Force Calculation ==
  note: Convert Sum of Moments to Local Coordinates
  note: Convert Equivalent Midpoint Couple to Local Coordinates
  note: Equivalent MP Couple
  note: Convert to Local Moment
  RWTorqueGlobal : Inport
  LWTorqueGlobal : Inport  Port=2
  LWForceGlobal : Inport  Port=3
  MPForceGlobal : Inport  Port=4
  RWForceGlobal : Inport  Port=5
  LeftWristPositionGlobal : Inport  Port=6
  MidpointPositionGlobal : Inport  Port=7
  RightWristPositionGlobal : Inport  Port=8
  ClubCOMPositionGlobal : Inport  Port=9
  Demux : Demux  Outputs=3
  Equivalent Midhands Couple Global : Sum  Inputs=+-
  Equivalent Midpoint Couple Local : Product  Multiplication=Matrix(*)
  LH MOFGlobal : matrix_library/Cross Product
  LHRVector : Sum  Inputs=+-
  LeftHandMOFLocal : Product  Multiplication=Matrix(*)
  MP MOF Global : matrix_library/Cross Product
  MPRVector : Sum  Inputs=+-
  MidpointMOFLocal : Product  Multiplication=Matrix(*)
  RH MOFGlobal : matrix_library/Cross Product
  RHRVector : Sum  Inputs=+-
  RightHandMOFLocal : Product  Multiplication=Matrix(*)
  RotationTransformLeftHand : nesl_utility/PS-Simulink Converter  PhysicalDomain=network_engine_domain  SubClassName=ps_output  LeftPortType=input  RightPortType=output  PseudoPeriodic=off  Frequencies=[]  VectorFormat=1-D array  Unit=inherit  AffineConversion=off
  RotationTransformMidpoint : nesl_utility/PS-Simulink Converter  PhysicalDomain=network_engine_domain  SubClassName=ps_output  LeftPortType=input  RightPortType=output  PseudoPeriodic=off  Frequencies=[]  VectorFormat=1-D array  Unit=inherit  AffineConversion=off
  RotationTransformMidpoint1 : nesl_utility/PS-Simulink Converter  PhysicalDomain=network_engine_domain  SubClassName=ps_output  LeftPortType=input  RightPortType=output  PseudoPeriodic=off  Frequencies=[]  VectorFormat=1-D array  Unit=inherit  AffineConversion=off
  RotationTransformMidpoint2 : nesl_utility/PS-Simulink Converter  PhysicalDomain=network_engine_domain  SubClassName=ps_output  LeftPortType=input  RightPortType=output  PseudoPeriodic=off  Frequencies=[]  VectorFormat=1-D array  Unit=inherit  AffineConversion=off
  RotationTransformRightHand : nesl_utility/PS-Simulink Converter  PhysicalDomain=network_engine_domain  SubClassName=ps_output  LeftPortType=input  RightPortType=output  PseudoPeriodic=off  Frequencies=[]  VectorFormat=1-D array  Unit=inherit  AffineConversion=off
  Sum of Moments Global : Sum  Inputs=++++
  SumofMomentsonClubLocal : Product  Multiplication=Matrix(*)
  Transform Sensor{,1..4} (5 alike) : sm_lib/Frames and Transforms/Transform Sensor  MeasurementFrame=World  RotationSequence=XYX  SenseAngle=off  SenseAxis=off  SenseQ=off  SenseR=on  SenseRotationSequence=off  SenseOmegaX=off  SenseOmegaY=off  SenseOmegaZ=off  SenseOmega=off  SenseQDot=off  SenseRDot=off  SenseRotationSequenceDot=off  SenseAlphaX=off  SenseAlphaY=off  SenseAlphaZ=off  SenseAlpha=off  SenseQDDot=off  SenseRDDot=off  SenseX=off  SenseY=off  SenseZ=off  SenseXYZ=off  SenseRad=off  SenseAzim=off  SenseDist=off  SenseInc=off  SenseXDot=off  SenseYDot=off  SenseZDot=off  SenseXYZDot=off  SenseRadDot=off  SenseAzimDot=off  SenseDistDot=off  SenseIncDot=off  SenseXDDot=off  SenseYDDot=off  SenseZDDot=off  SenseXYZDDot=off  SenseRadDDot=off  SenseAzimDDot=off  SenseDistDDot=off  SenseIncDDot=off
  World Frame : sm_lib/Frames and Transforms/World Frame
  LeftWrist : PMIOPort  Side=Left
  Midpoint : PMIOPort  Port=2  Side=Left
  RightWrist : PMIOPort  Port=3  Side=Left
  LWMOFonClub : Outport
  RWMOFonClub : Outport  Port=2
  wires:
  RHRVector/1 -> RH MOFGlobal/1
  LHRVector/1 -> LH MOFGlobal/1
  LWForceGlobal/1 -> LH MOFGlobal/2
  LeftWristPositionGlobal/1 -> LHRVector/1
  ClubCOMPositionGlobal/1 -> RHRVector/2, MPRVector/2, LHRVector/2
  MidpointPositionGlobal/1 -> MPRVector/1
  RightWristPositionGlobal/1 -> RHRVector/1
  LH MOFGlobal/1 -> LWMOFonClub/1, Sum of Moments Global/1, LeftHandMOFLocal/2  "LHMOFonClubGlobal"
  MP MOF Global/1 -> Equivalent Midhands Couple Global/2, MidpointMOFLocal/2  "MPMOFonClubGlobal"
  RH MOFGlobal/1 -> Sum of Moments Global/2, RWMOFonClub/1, RightHandMOFLocal/2  "RHMOFonClubGlobal"
  MPForceGlobal/1 -> MP MOF Global/2
  MPRVector/1 -> MP MOF Global/1
  RWForceGlobal/1 -> RH MOFGlobal/2
  RotationTransformRightHand/1 -> RightHandMOFLocal/1
  RotationTransformMidpoint/1 -> MidpointMOFLocal/1
  RotationTransformLeftHand/1 -> LeftHandMOFLocal/1
  Equivalent Midhands Couple Global/1 -> Equivalent Midpoint Couple Local/2  "EquivalentMidpointCoupleGlobal"
  LWTorqueGlobal/1 -> Sum of Moments Global/3
  RWTorqueGlobal/1 -> Sum of Moments Global/4
  Sum of Moments Global/1 -> SumofMomentsonClubLocal/2, Equivalent Midhands Couple Global/1  "SumofMomentsonClubGlobal"
  RotationTransformMidpoint1/1 -> Equivalent Midpoint Couple Local/1
  RotationTransformMidpoint2/1 -> SumofMomentsonClubLocal/1
  Equivalent Midpoint Couple Local/1 -> Demux/1  "EquivalentMidpointCoupleLocal"
  connections:
  RightWrist/RConn1 -- Transform Sensor2/LConn1
  LeftWrist/RConn1 -- Transform Sensor/LConn1
  RotationTransformRightHand/LConn1 -- Transform Sensor2/RConn2
  RotationTransformMidpoint/LConn1 -- Transform Sensor1/RConn2
  RotationTransformLeftHand/LConn1 -- Transform Sensor/RConn2
  World Frame/RConn1 -- Transform Sensor3/RConn1 -- Transform Sensor1/RConn1 -- Transform Sensor2/RConn1 -- Transform Sensor/RConn1 -- Transform Sensor4/RConn1
  RotationTransformMidpoint1/LConn1 -- Transform Sensor3/RConn2
  Midpoint/RConn1 -- Transform Sensor3/LConn1 -- Transform Sensor4/LConn1 -- Transform Sensor1/LConn1
  RotationTransformMidpoint2/LConn1 -- Transform Sensor4/RConn2
